simulink model "pos_att"  (R2019a)
settings: Solver=VariableStepAuto  StartTime=0.0  StopTime=20  RelTol=1e-3
values from neighbouring files (symbols this model uses):
  A_ad = [zeros(3,3), eye(3) ... (first row only)    [admittance.m]
  Ak = zeros(18,18)    [Kalman_filter.m]
  B_ad = [zeros(3,3), zeros(3,3) ... (first row only)    [admittance.m]
  Bk = zeros(18,4)    [Kalman_filter.m]
  C_ad = [eye(3), zeros(3,3)]    [admittance.m]
  Ck = zeros(6,18)    [Kalman_filter.m]
  D_ad = zeros(3,6)    [admittance.m]
  Dk = zeros(6,4)    [Kalman_filter.m]
  V = 10*eye(6)    [Kalman_filter.m]
undefined symbols (not defined in the file or in its folder): A, B, C, Continuous, D, init_state, Time
libraries: ctrlSharedLib x1
settings Model: Creator=anagh  LastModifiedBy=anagh

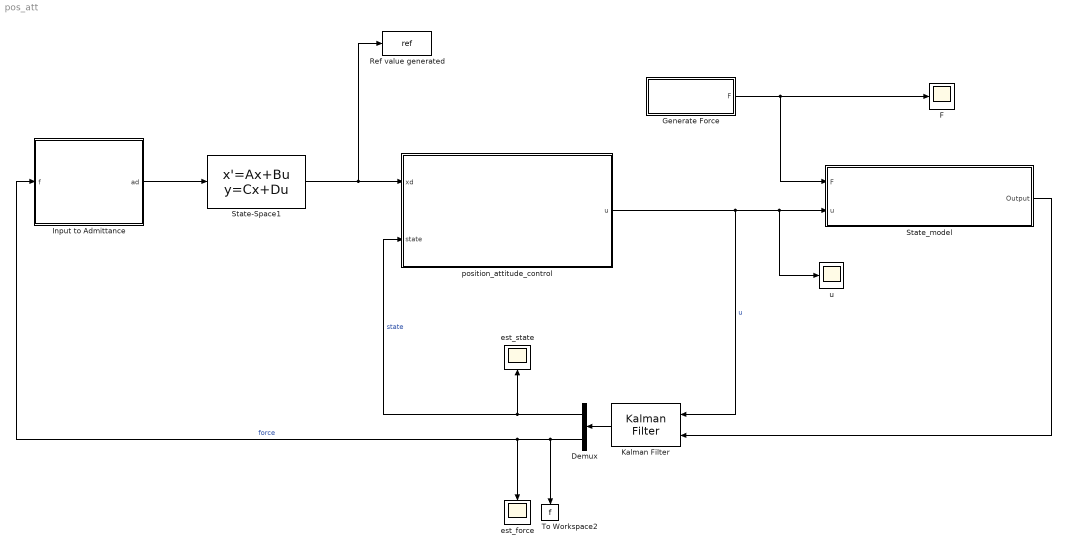
== system pos_att ==
  " Input to Admittance " : MATLAB Function  TreatAsAtomicUnit=on
  Demux : Demux  Outputs=[15, 3]
  F : Scope
  Generate Force : Subsystem
  "Kalman Filter " : ctrlSharedLib/Kalman Filter  TimeDomain=Continuous-Time  UseCurrentEstimator=on  ModelSource=Individual A, B, C, D matrices  ModelSourceVariable=ss(0.95,1,1,0,1)  A=Ak  B=Bk  C=Ck  D=Dk  NumberOfStates=1  NumberOfInputs=1  NumberOfOutputs=1  InitialEstimateSource=Dialog  X0=0  P0=10  UseK=off  UseGH=off  NumberOfProcessNoiseInputs=1  G=1  TimeInvariantG=on  H=0  TimeInvariantH=on  Q=W  TimeInvariantQ=on  R=V  TimeInvariantR=on  N=0  TimeInvariantN=on  AddInputPort=on  AddEnablePort=off  OutputEstimatedY=off  OutputP=off  Ts=-1
      settings: SourceProductBaseCode=CT
  Ref value generated : ToWorkspace  VariableName=ref  SaveFormat=Structure With Time  SampleTime=-1
  State-Space1 : StateSpace  A=A_ad  B=B_ad  C=C_ad  D=D_ad  InitialCondition=[0 0 0 0 0 0]
  State_model : Subsystem
  To Workspace2 : ToWorkspace  VariableName=f  SaveFormat=Structure With Time  SampleTime=-1
  est_force : Scope
  est_state : Scope
  position_attitude_control : MATLAB Function  TreatAsAtomicUnit=on
  "u " : Scope
  wires:
  "Kalman Filter "/1 -> Demux/1
  Demux/2 -> " Input to Admittance "/1(f), est_force/1, To Workspace2/1  "force"
  Demux/1 -> position_attitude_control/2(state), est_state/1  "state"
  " Input to Admittance "/1(ad) -> State-Space1/1
  State-Space1/1 -> Ref value generated/1, position_attitude_control/1(xd)
  Generate Force/1(F) -> State_model/1(F), F/1
  State_model/1(Output) -> "Kalman Filter "/2
  position_attitude_control/1(u) -> "Kalman Filter "/1, "u "/1, State_model/2("u ")  "u"

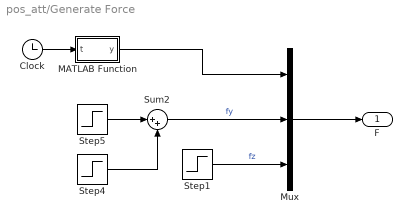
== system pos_att/Generate Force ==
  Clock : Clock
  MATLAB Function : MATLAB Function  TreatAsAtomicUnit=on
  Mux : Mux  Inputs=3
  Step1 : Step  After=0  SampleTime=0
  Step4 : Step  Time=6  After=0  SampleTime=0
  Step5 : Step  After=0  SampleTime=0
  Sum2 : Sum  Inputs=|++
  F : Outport
  wires:
  Step5/1 -> Sum2/1
  Sum2/1 -> Mux/2  "fy"
  Step4/1 -> Sum2/2
  Mux/1 -> F/1
  Step1/1 -> Mux/3  "fz"
  Clock/1 -> MATLAB Function/1(t)
  MATLAB Function/1(y) -> Mux/1

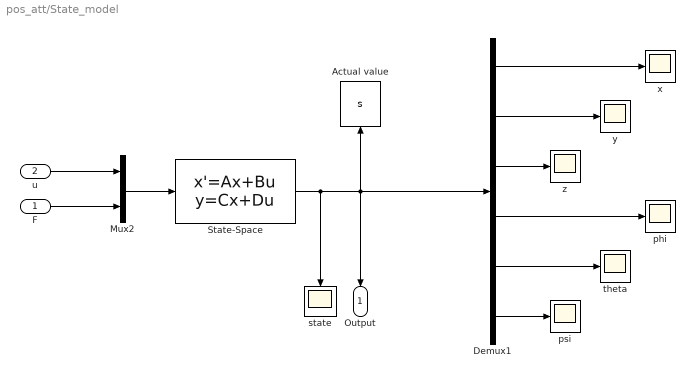
== system pos_att/State_model ==
  F : Inport
  "u " : Inport  Port=2
  " Actual value" : ToWorkspace  VariableName=s  SaveFormat=Structure With Time  SampleTime=-1
  Demux1 : Demux  Outputs=6
  Mux2 : Mux  Inputs=2
  State-Space : StateSpace  A=A  B=B  C=C  D=D  InitialCondition=init_state
  phi : Scope
  psi : Scope
  state : Scope
  theta : Scope
  "x " : Scope
  y : Scope
  z : Scope
  Output : Outport
  wires:
  Demux1/4 -> phi/1
  "u "/1 -> Mux2/1
  Demux1/6 -> psi/1
  F/1 -> Mux2/2
  Demux1/2 -> y/1
  Demux1/1 -> "x "/1
  Demux1/3 -> z/1
  Demux1/5 -> theta/1
  State-Space/1 -> Demux1/1, " Actual value"/1, Output/1, state/1
  Mux2/1 -> State-Space/1

== matlab function pos_att/ Input to Admittance  ==
  data: ad output; f input
function ad = Input_desired(f)

x_d = 1;
y_d = 1;
z_d = 5;

fx = f(1);

fy = f(2);

fz = f(3);

ad = [x_d, y_d, z_d, fx, fy, fz]';

== matlab function pos_att/position_attitude_control ==
  data: xd input; u output; state input
function u = Position_attitude_control(xd, state)
g = 9.81;   % [ms^-2]
Ix = 0.5;   % [kg*m^2]
Iy = 0.5;
Iz = 0.9;
Ir = 0.005;
Om_r = 70;  % [s^-2]
m = 2;      % [kg]
l = 0.25;   % [m]
d = 0.03;
m1 = 0.1;
T1 = 0.001;
T2 = 0.001;

% State

x = state(1);
y = state(2);
z = state(3);
vx = state(4);
vy = state(5);
vz = state(6);
phi = state(7);
theta = state(8);
psi = state(9);
phi_dot = state(10);
theta_dot = state(11);
psi_dot = state(12);
tau_phi = state(13);
tau_theta = state(14);
tau_psi = state(15);

% Controller Gains 

%  kxp=3.5; kxd=0.89;
%  kyp=3.45; kyd=0.899;
%  kzp=18; kzd=6; 
%  kthp=20; kthd=3;
%  kphp=20; kphd=3;
%  ktsp=1; ktsd=1;

kxp=7; kxd=1.78;
 kyp=3.45; kyd=0.899;
 kzp=18; kzd=6; 
 kthp=40; kthd=6;
 kphp=20; kphd=3;
 ktsp=1; ktsd=1;

% Reference Trajectory
 
x_d = xd(1);
y_d = xd(2);
z_d = xd(3);

vx_d = 0;
vy_d = 0;
vz_d = 0;

%Controller
theta_r = -1/9.8*(kxp*(x_d-state(1,1)+kxd*(0-state(4,1))));
phi_r = 1/9.8*(kyp*(y_d-state(2,1)+kyd*(0-state(5,1))));
    
T = -m*(kzp*(z_d-state(3,1))+kzd*(0-state(6,1))); 
psi_cmd = ktsp*(0-state(9,1))+ktsd*(0-state(12,1));
phi_cmd = kphp*(phi_r-state(7,1))+kphd*(0-state(10,1));
theta_cmd = kthp*(theta_r-state(8,1))+kthd*(0-state(11,1));
    
u = [T, phi_cmd, theta_cmd, psi_cmd]';

== matlab function pos_att/Generate Force/MATLAB Function ==
  data: t input; y output
function y = fcn(t)
% if t > 1 && t < 1.5
%     fx=1;
% else
%     fx=0;
% end

y = sin(t);
